simulink model "sin_wave_demodulate"  (R2023b)
settings: Solver=VariableStepAuto  StartTime=0.0  StopTime=0.15  RelTol=1e-3
PreLoadFcn:
  | clear all;
  | 
  | fs = 1e6
InitFcn:
  | fs = 1e6
libraries: hdlBasic x33, hdlsllib x3, dspsrcs4 x2, simulink x1, vmcUtilities x1
settings Model: Creator=David Northcote  LastModifiedBy=clb20123
settings SolverCC: AlgebraicLoopSolver=TrustRegion
settings DataIOCC: ReturnWorkspaceOutputs=off
settings DebuggingCC: UnconnectedInputMsg=warning  UnconnectedOutputMsg=warning  UnconnectedLineMsg=warning  ArithmeticOperatorsInVariantConditions=warning
settings ModelReferenceCC: EnableRefExpFcnMdlSchedulingChecks=on
settings SFSimCC: SimUseLocalCustomCode=off  CustomCodeUndefinedFunction=UseInterfaceOnly
settings RTWCC: RTWUseLocalCustomCode=off

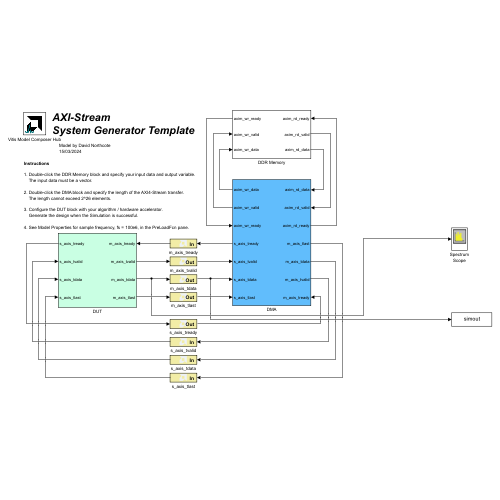
[thumbnail: Simulink's stored preview of the top-level diagram]
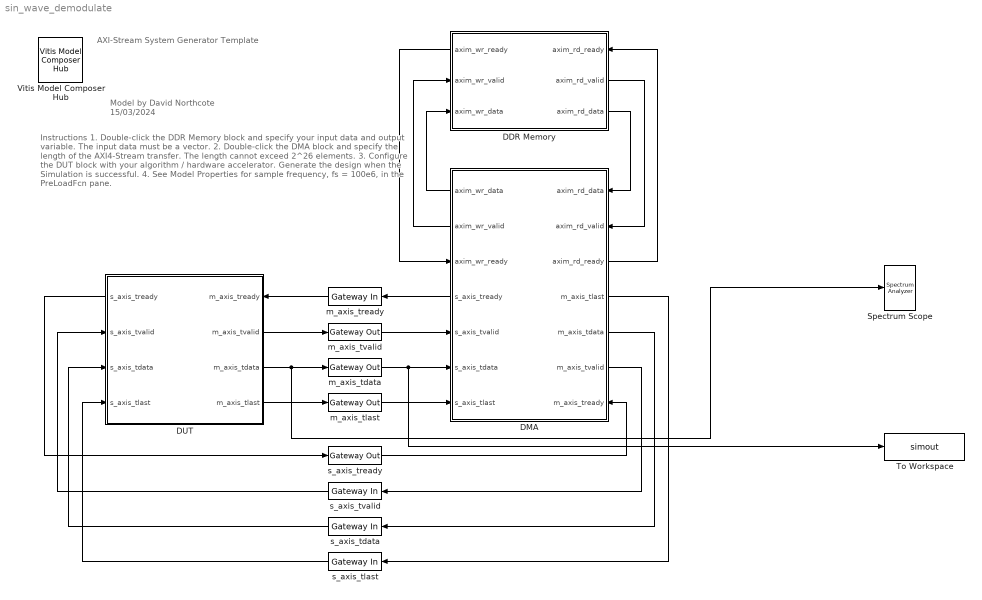
== system sin_wave_demodulate ==
  note: Instructions
      |
      | 1. Double-click the DDR Memory block and specify your input data and output variable.
      | The input data must be a vector.
      |
      | 2. Double-click the DMA block and specify the length of the AXI4-Stream transfer.
      | The length cannot exceed 2^26 elements.
      |
      | 3. Configure the DUT block with your algorithm / hardware accelerator.
      | Generate the design when the Simulation is successful.
      |
      | 4. See Model Properties for sample frequency, fs = 100e6, in the PreLoadFcn pane.
  note: Model by David Northcote
      | 15/03/2024
  note: AXI-Stream
      | System Generator Template
  DDR Memory : Subsystem  mask{bufferOut=[1 1 1 1 1 1 1 1 1 1 1 1 1 1], dtype=uint32, outVar='bufferIn'}
      mask prompts: bufferOut "Data to be sent:"; dtype "Data type:"; outVar "Output variable name:"
      mask init:
      | dtypeStr = get_param(gcb, 'dtype');
      | outVarStr = get_param(gcb, 'outVar');
      | set_param([gcb, '/Buffer In/To Workspace'], 'VariableName', outVar)
      settings: PortSchema="{\"entries\":[{\"content\":{\"sides\":[{\"content\":{\"connectorIds\":[\"Out3\",\"In1\",\"In2\"]},\"type\":\"ConnectorPlacement.EquallySpacedRectSide\",\"uuid\":\"10820561-fcd3-42da-ac38-14c6f993f770\"},{\"content\":{\"connectorIds\":[\"In3\",\"Out1\",\"Out2\"],\"side\":\"RIGHT\"},\"type\":\"ConnectorPlacement.EquallySpacedRectSide\",\"uuid\":\"072276f7-1cf8-495f-bb0a-1bca7e8326ea\"},{\"content\":{\"connectorIds\":[],\"side\":\"TOP\"},\"type\":\"ConnectorPlacement.EquallySpacedRectSide\",\"uuid\":\"f5b81d71-f8e7-451c-95ca-ef44dafc9f7a\"}]},\"type\":\"ConnectorPlacement.EquallySpacedConnector\",\"uuid\":\"59ea238c-ea64-4381-b9ec-a479227d5ff5\"}],\"packageUris\":[\"http://schema.mathworks.com/mf0/Connector/19700101\"],\"version\":\"1.0\"}"
      mask TypeOptions dtype: uint32 | int32
      mask DialogControl DescGroupVar Prompt: DDR Memory
      mask DialogControl DescTextVar Prompt: Block simulating a DDR memory controller.
      mask DialogControl ParameterGroupVar Prompt: MM2S
      mask DialogControl Container4 Prompt: S2MM
  DMA : Subsystem  mask{N=32}
      mask prompts: N "Length of data:"
      settings: PortSchema="{\"entries\":[{\"content\":{\"sides\":[{\"content\":{\"connectorIds\":[\"Out5\",\"Out6\",\"In1\",\"Out7\",\"In2\",\"In3\",\"In4\"]},\"type\":\"ConnectorPlacement.EquallySpacedRectSide\",\"uuid\":\"c102abcb-2e00-4fd7-85df-5b9b0b898bd0\"},{\"content\":{\"connectorIds\":[\"In5\",\"In6\",\"Out1\",\"Out2\",\"Out3\",\"Out4\",\"In7\"],\"side\":\"RIGHT\"},\"type\":\"ConnectorPlacement.EquallySpacedRectSide\",\"uuid\":\"9e178eef-1e1d-41e3-971e-2eb7c6a5387e\"},{\"content\":{\"connectorIds\":[],\"side\":\"TOP\"},\"type\":\"ConnectorPlacement.EquallySpacedRectSide\",\"uuid\":\"12cf59e0-f07a-41d8-b174-5a1eb72b1624\"},{\"content\":{\"connectorIds\":[],\"side\":\"BOTTOM\"},\"type\":\"ConnectorPlacement.EquallySpacedRectSide\",\"uuid\":\"a47cc6bb-72ec-4c9c-b625-c22428f6e2e0\"}]},\"type\":\"ConnectorPlacement.EquallySpacedConnector\",\"uuid\":\"cad21ed4-9065-49eb-a891-849a058d114a\"}],\"packageUris\":[\"http://schema.mathworks.com/mf0/Connector/19700101\"],\"version\":\"1.0\"}"
      mask DialogControl DescGroupVar Prompt: AXI DMA
      mask DialogControl DescTextVar Prompt: Block simulating an AXI DMA.
      mask DialogControl ParameterGroupVar Prompt: Main
  DUT : Subsystem
      settings: PortSchema="{\"entries\":[{\"content\":{\"sides\":[{\"content\":{\"connectorIds\":[\"Out4\",\"In1\",\"In2\",\"In3\"]},\"type\":\"ConnectorPlacement.EquallySpacedRectSide\",\"uuid\":\"c102abcb-2e00-4fd7-85df-5b9b0b898bd0\"},{\"content\":{\"connectorIds\":[\"In4\",\"Out1\",\"Out2\",\"Out3\"],\"side\":\"RIGHT\"},\"type\":\"ConnectorPlacement.EquallySpacedRectSide\",\"uuid\":\"9e178eef-1e1d-41e3-971e-2eb7c6a5387e\"},{\"content\":{\"connectorIds\":[],\"side\":\"TOP\"},\"type\":\"ConnectorPlacement.EquallySpacedRectSide\",\"uuid\":\"12cf59e0-f07a-41d8-b174-5a1eb72b1624\"}]},\"type\":\"ConnectorPlacement.EquallySpacedConnector\",\"uuid\":\"cad21ed4-9065-49eb-a891-849a058d114a\"}],\"packageUris\":[\"http://schema.mathworks.com/mf0/Connector/19700101\"],\"version\":\"1.0\"}"
  Spectrum Scope : SpectrumAnalyzer  WindowPosition=[182.000000,-8.000000,1444.000000,881.000000,]  ScopeFrameLocation=window  SpectrumType=Power density  Method=Welch  SampleRate=48000  PlotAsTwoSidedSpectrum=off  AxesScaling=Manual  FrequencySpan=Start and stop frequencies  Span=24000  CenterFrequency=12000  StartFrequency=0  StopFrequency=fs/2  FrequencyResolutionMethod=Window length  FFTLengthSource=Property  FFTLength=2048  WindowLength=2048  OverlapPercent=50  AveragingMethod=Running  SpectralAverages=2  SpectrumUnits=dBW/Hz  YLabel=Magnitude  YLimits=[-1013.06950271,305.05930835]  SelectedToolstripTab=spectrumAnalyzerToolstrip.measurementsTab  DefaultConfigurationName=spbscopes.SpectrumAnalyzerBlockCfg  IsFrequencyInputMode=0  FrequencyVectorPort=0  FrequencyVectorFromPort=0  FrequencyInputRBWPort=0  FrequencyInputRBWFromPort=0  SegLen=2048
  To Workspace : ToWorkspace  VariableName=simout  SaveFormat=Timeseries  SampleTime=-1
  Vitis Model Composer Hub : vmcUtilities/Vitis Model Composer Hub  Tag=genX  CodeGeneration=off  SubsystemName=sin_wave_modulate  CompilationType=HDLCompilation  ExportTypeV2=IP Catalog  TargetDirectory=./netlist  exportDesign=on  analyzeDesign=off  validateDesignOnHw=off  ExportType=System Generator  IpVendor=xilinx.com  IpLibrary=hls  IpVersion=1.0  IpHWLanguage=Verilog  AieCompilerOptions={}  AieSimulatorOptions={}  CreateTestbench=off  TestbenchStackSize=10  RunRtlSim=off  RunCSim=off  RunAieSim=off  AieSimTimeout=50000  RunAieSimProfiling=off  LaunchVitisAnalyzer=off  PlotOutput=off  RunX86Sim=off  X86SimTimeout=10  GenHwImage=off  GenLibadfXo=on  GenHwValidationCode=off  PlatformType=Not Specified  HwSystemType=Baremetal  HwValidationTarget=hw  ProjDevice=xczu43dr-ffve1156-2-e  ProjDevicePart=xczu43dr-ffve1156-2-e  SamplePeriod=-1  ClockFrequency=200  DataPathParallelism=1  xilinxfamily=zynquplusRFSOC  part=xczu43dr  speed=-2-e  package=ffve1156  directory=./netlist\ip\sin_wave_modulate\src  testbench=off  incr_netlist=off  synthesis_tool=Vivado  clock_wrapper=Clock Enables  dbl_ovrd=According to Block Masks  dcm_input_clock_period=10  sysclk_period=10  simulink_period=1/fs  eval_field=0  IPInfoJsonString="{\"HDLSubsystem\":{\"SubsystemName\":\"AXI_Overtone\",\"IPName\":\"axi_stream_template\",\"IPLibrary\":\"SysGen\",\"IPVendor\":\"strath.ac.uk\",\"IPVersion\":\"1.0\",\"TargetDirectory\":\"./netlist\",\"SubsystemDir\":\"./netlist\\\\ip\\\\AXI_Overtone\"},\"SubsystemTag\":\"HDLNode\"}"  LogFileName=''  NThreads=4
  m_axis_tdata : hdlBasic/Gateway Out  inherit_from_input=on  hdl_port=on  rows=1  columns=1  UseAsDAC=off  DACChannel='1'  interface=None  automatic_assignment=on  address_offset=hex2dec('00')  intf_name=''  intf_description=''  timing_constraint=None  locs_specified=off  LOCs={}  io_standard={}  XmcBlockStatus=1  maskContainerNames=group4  block_type=gatewayout  block_config=sysgen:gateway_out_config  block_width_w=590  block_height_w=620  block_width=620  block_height=750
  m_axis_tlast : hdlBasic/Gateway Out  inherit_from_input=on  hdl_port=on  rows=1  columns=1  UseAsDAC=off  DACChannel='1'  interface=None  automatic_assignment=on  address_offset=hex2dec('00')  intf_name=''  intf_description=''  timing_constraint=None  locs_specified=off  LOCs={}  io_standard={}  XmcBlockStatus=1  maskContainerNames=group4  block_type=gatewayout  block_config=sysgen:gateway_out_config  block_width_w=590  block_height_w=620  block_width=620  block_height=750
  m_axis_tready : hdlBasic/Gateway In  gui_display_data_type=Boolean  arith_type=Boolean  n_bits=16  bin_pt=14  preci_type=Single  exp_width=8  frac_width=24  rows=1  columns=1  quantization="Round  (unbiased: +/- Inf)"  overflow=Saturate  period=1/fs  UseAsADC=off  ADCChannel='1'  interface=None  automatic_assignment=on  address_offset=hex2dec('00')  intf_name=''  intf_description=''  default_value=0  timing_constraint=None  locs_specified=off  LOCs={}  io_standard={}  inherit_from_input=off  hdl_port=on  XmcBlockStatus=1  maskContainerNames=group4  block_type=gatewayin  block_config=sysgen:gateway_in_config  block_width_w=590  block_height_w=620  block_width=640  block_height=850
  m_axis_tvalid : hdlBasic/Gateway Out  inherit_from_input=on  hdl_port=on  rows=1  columns=1  UseAsDAC=off  DACChannel='1'  interface=None  automatic_assignment=on  address_offset=hex2dec('00')  intf_name=''  intf_description=''  timing_constraint=None  locs_specified=off  LOCs={}  io_standard={}  XmcBlockStatus=1  maskContainerNames=group4  block_type=gatewayout  block_config=sysgen:gateway_out_config  block_width_w=590  block_height_w=620  block_width=620  block_height=750
  s_axis_tdata : hdlBasic/Gateway In  gui_display_data_type=Fixed-point  arith_type=Unsigned  n_bits=1  bin_pt=0  preci_type=Single  exp_width=8  frac_width=24  rows=1  columns=1  quantization="Round  (unbiased: +/- Inf)"  overflow=Saturate  period=1/fs  UseAsADC=off  ADCChannel='1'  interface=None  automatic_assignment=on  address_offset=hex2dec('00')  intf_name=''  intf_description=''  default_value=0  timing_constraint=None  locs_specified=off  LOCs={}  io_standard={}  inherit_from_input=off  hdl_port=on  XmcBlockStatus=1  maskContainerNames=group4  block_type=gatewayin  block_config=sysgen:gateway_in_config  block_width_w=590  block_height_w=620  block_width=640  block_height=850
  s_axis_tlast : hdlBasic/Gateway In  gui_display_data_type=Boolean  arith_type=Boolean  n_bits=16  bin_pt=14  preci_type=Single  exp_width=8  frac_width=24  rows=1  columns=1  quantization="Round  (unbiased: +/- Inf)"  overflow=Saturate  period=1/fs  UseAsADC=off  ADCChannel='1'  interface=None  automatic_assignment=on  address_offset=hex2dec('00')  intf_name=''  intf_description=''  default_value=0  timing_constraint=None  locs_specified=off  LOCs={}  io_standard={}  inherit_from_input=off  hdl_port=on  XmcBlockStatus=1  maskContainerNames=group4  block_type=gatewayin  block_config=sysgen:gateway_in_config  block_width_w=590  block_height_w=620  block_width=640  block_height=850
  s_axis_tready : hdlBasic/Gateway Out  inherit_from_input=on  hdl_port=on  rows=1  columns=1  UseAsDAC=off  DACChannel='1'  interface=None  automatic_assignment=on  address_offset=hex2dec('00')  intf_name=''  intf_description=''  timing_constraint=None  locs_specified=off  LOCs={}  io_standard={}  XmcBlockStatus=1  maskContainerNames=group4  block_type=gatewayout  block_config=sysgen:gateway_out_config  block_width_w=590  block_height_w=620  block_width=620  block_height=750
  s_axis_tvalid : hdlBasic/Gateway In  gui_display_data_type=Boolean  arith_type=Boolean  n_bits=16  bin_pt=14  preci_type=Single  exp_width=8  frac_width=24  rows=1  columns=1  quantization="Round  (unbiased: +/- Inf)"  overflow=Saturate  period=1/fs  UseAsADC=off  ADCChannel='1'  interface=None  automatic_assignment=on  address_offset=hex2dec('00')  intf_name=''  intf_description=''  default_value=0  timing_constraint=None  locs_specified=off  LOCs={}  io_standard={}  inherit_from_input=off  hdl_port=on  XmcBlockStatus=1  maskContainerNames=group4  block_type=gatewayin  block_config=sysgen:gateway_in_config  block_width_w=590  block_height_w=620  block_width=640  block_height=850
  wires:
  s_axis_tvalid/1 -> DUT/1(s_axis_tvalid)
  s_axis_tdata/1 -> DUT/2(s_axis_tdata)
  s_axis_tlast/1 -> DUT/3(s_axis_tlast)
  m_axis_tready/1 -> DUT/4(m_axis_tready)
  DUT/4(s_axis_tready) -> s_axis_tready/1
  DUT/2(m_axis_tdata) -> Spectrum Scope/1, m_axis_tdata/1
  DUT/1(m_axis_tvalid) -> m_axis_tvalid/1
  DUT/3(m_axis_tlast) -> m_axis_tlast/1
  s_axis_tready/1 -> DMA/7(m_axis_tready)
  DMA/4(m_axis_tvalid) -> s_axis_tvalid/1
  DMA/3(m_axis_tdata) -> s_axis_tdata/1
  DMA/2(m_axis_tlast) -> s_axis_tlast/1
  DMA/7(s_axis_tready) -> m_axis_tready/1
  m_axis_tvalid/1 -> DMA/2(s_axis_tvalid)
  m_axis_tdata/1 -> To Workspace/1, DMA/3(s_axis_tdata)
  m_axis_tlast/1 -> DMA/4(s_axis_tlast)
  DMA/1(axim_rd_ready) -> DDR Memory/3(axim_rd_ready)
  DDR Memory/1(axim_rd_valid) -> DMA/6(axim_rd_valid)
  DDR Memory/2(axim_rd_data) -> DMA/5(axim_rd_data)
  DDR Memory/3(axim_wr_ready) -> DMA/1(axim_wr_ready)
  DMA/6(axim_wr_valid) -> DDR Memory/1(axim_wr_valid)
  DMA/5(axim_wr_data) -> DDR Memory/2(axim_wr_data)

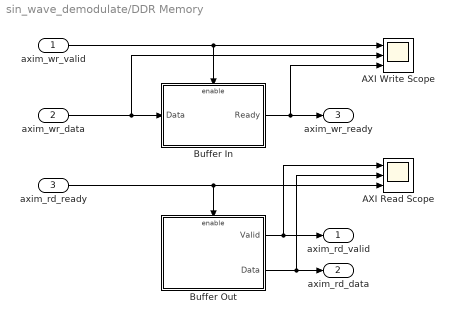
== system sin_wave_demodulate/DDR Memory ==
  axim_wr_valid : Inport
  axim_wr_data : Inport  Port=2
  axim_rd_ready : Inport  Port=3
  AXI Read Scope : Scope  NumInputPorts=3
  AXI Write Scope : Scope  NumInputPorts=3
  Buffer In : Subsystem
  Buffer Out : Subsystem
  axim_rd_valid : Outport
  axim_rd_data : Outport  Port=2
  axim_wr_ready : Outport  Port=3
  wires:
  Buffer Out/1(Valid) -> AXI Read Scope/1, axim_rd_valid/1
  Buffer Out/2(Data) -> AXI Read Scope/2, axim_rd_data/1
  axim_rd_ready/1 -> Buffer Out/Enable, AXI Read Scope/3
  axim_wr_data/1 -> AXI Write Scope/2, Buffer In/1(Data)
  Buffer In/1(Ready) -> AXI Write Scope/3, axim_wr_ready/1
  axim_wr_valid/1 -> Buffer In/Enable, AXI Write Scope/1

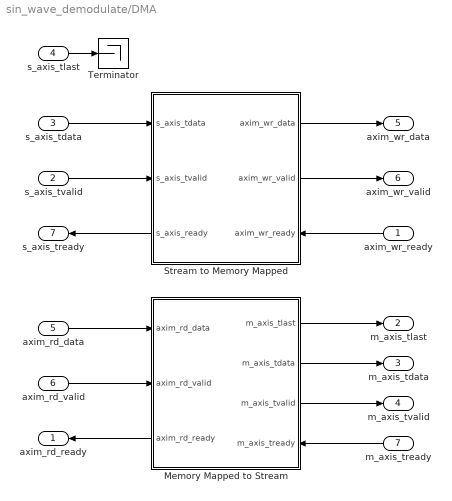
== system sin_wave_demodulate/DMA ==
  axim_wr_ready : Inport
  s_axis_tvalid : Inport  Port=2
  s_axis_tdata : Inport  Port=3
  s_axis_tlast : Inport  Port=4
  axim_rd_data : Inport  Port=5
  axim_rd_valid : Inport  Port=6
  m_axis_tready : Inport  Port=7
  Memory Mapped to Stream : Subsystem
      settings: PortSchema="{\"entries\":[{\"content\":{\"sides\":[{\"content\":{\"connectorIds\":[\"In1\",\"In2\",\"Out4\"]},\"type\":\"ConnectorPlacement.EquallySpacedRectSide\",\"uuid\":\"10820561-fcd3-42da-ac38-14c6f993f770\"},{\"content\":{\"connectorIds\":[\"Out1\",\"Out2\",\"Out3\",\"In3\"],\"side\":\"RIGHT\"},\"type\":\"ConnectorPlacement.EquallySpacedRectSide\",\"uuid\":\"072276f7-1cf8-495f-bb0a-1bca7e8326ea\"},{\"content\":{\"connectorIds\":[],\"side\":\"TOP\"},\"type\":\"ConnectorPlacement.EquallySpacedRectSide\",\"uuid\":\"f5b81d71-f8e7-451c-95ca-ef44dafc9f7a\"}]},\"type\":\"ConnectorPlacement.EquallySpacedConnector\",\"uuid\":\"59ea238c-ea64-4381-b9ec-a479227d5ff5\"}],\"packageUris\":[\"http://schema.mathworks.com/mf0/Connector/19700101\"],\"version\":\"1.0\"}"
  Stream to Memory Mapped : Subsystem
      settings: PortSchema="{\"entries\":[{\"content\":{\"sides\":[{\"content\":{\"connectorIds\":[\"In1\",\"In2\",\"Out3\"]},\"type\":\"ConnectorPlacement.EquallySpacedRectSide\",\"uuid\":\"10820561-fcd3-42da-ac38-14c6f993f770\"},{\"content\":{\"connectorIds\":[\"Out1\",\"Out2\",\"In3\"],\"side\":\"RIGHT\"},\"type\":\"ConnectorPlacement.EquallySpacedRectSide\",\"uuid\":\"072276f7-1cf8-495f-bb0a-1bca7e8326ea\"},{\"content\":{\"connectorIds\":[],\"side\":\"TOP\"},\"type\":\"ConnectorPlacement.EquallySpacedRectSide\",\"uuid\":\"f5b81d71-f8e7-451c-95ca-ef44dafc9f7a\"}]},\"type\":\"ConnectorPlacement.EquallySpacedConnector\",\"uuid\":\"59ea238c-ea64-4381-b9ec-a479227d5ff5\"}],\"packageUris\":[\"http://schema.mathworks.com/mf0/Connector/19700101\"],\"version\":\"1.0\"}"
  Terminator : Terminator
  axim_rd_ready : Outport
  m_axis_tlast : Outport  Port=2  VectorParamsAs1DForOutWhenUnconnected=off
  m_axis_tdata : Outport  Port=3  VectorParamsAs1DForOutWhenUnconnected=off
  m_axis_tvalid : Outport  Port=4  VectorParamsAs1DForOutWhenUnconnected=off
  axim_wr_data : Outport  Port=5
  axim_wr_valid : Outport  Port=6
  s_axis_tready : Outport  Port=7  VectorParamsAs1DForOutWhenUnconnected=off
  wires:
  m_axis_tready/1 -> Memory Mapped to Stream/3(m_axis_tready)
  Memory Mapped to Stream/1(m_axis_tlast) -> m_axis_tlast/1
  Memory Mapped to Stream/2(m_axis_tdata) -> m_axis_tdata/1
  Memory Mapped to Stream/3(m_axis_tvalid) -> m_axis_tvalid/1
  s_axis_tvalid/1 -> Stream to Memory Mapped/2(s_axis_tvalid)
  s_axis_tdata/1 -> Stream to Memory Mapped/1(s_axis_tdata)
  Stream to Memory Mapped/3(s_axis_ready) -> s_axis_tready/1
  s_axis_tlast/1 -> Terminator/1
  Stream to Memory Mapped/1(axim_wr_data) -> axim_wr_data/1
  Stream to Memory Mapped/2(axim_wr_valid) -> axim_wr_valid/1
  axim_wr_ready/1 -> Stream to Memory Mapped/3(axim_wr_ready)
  Memory Mapped to Stream/4(axim_rd_ready) -> axim_rd_ready/1
  axim_rd_data/1 -> Memory Mapped to Stream/1(axim_rd_data)
  axim_rd_valid/1 -> Memory Mapped to Stream/2(axim_rd_valid)

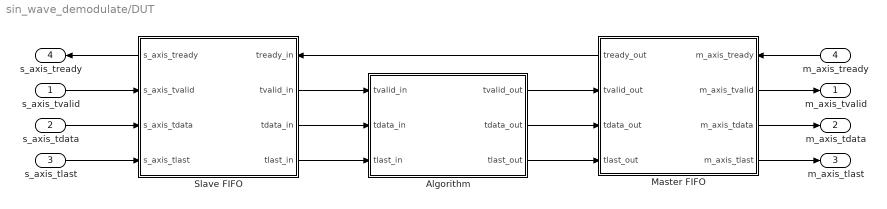
== system sin_wave_demodulate/DUT ==
  s_axis_tvalid : Inport
  s_axis_tdata : Inport  Port=2
  s_axis_tlast : Inport  Port=3
  m_axis_tready : Inport  Port=4
  Algorithm : Subsystem
  Master FIFO : Subsystem
      settings: PortSchema="{\"entries\":[{\"content\":{\"sides\":[{\"content\":{\"connectorIds\":[\"Out4\",\"In1\",\"In2\",\"In3\"]},\"type\":\"ConnectorPlacement.EquallySpacedRectSide\",\"uuid\":\"10820561-fcd3-42da-ac38-14c6f993f770\"},{\"content\":{\"connectorIds\":[\"In4\",\"Out1\",\"Out2\",\"Out3\"],\"side\":\"RIGHT\"},\"type\":\"ConnectorPlacement.EquallySpacedRectSide\",\"uuid\":\"072276f7-1cf8-495f-bb0a-1bca7e8326ea\"},{\"content\":{\"connectorIds\":[],\"side\":\"TOP\"},\"type\":\"ConnectorPlacement.EquallySpacedRectSide\",\"uuid\":\"f5b81d71-f8e7-451c-95ca-ef44dafc9f7a\"}]},\"type\":\"ConnectorPlacement.EquallySpacedConnector\",\"uuid\":\"59ea238c-ea64-4381-b9ec-a479227d5ff5\"}],\"packageUris\":[\"http://schema.mathworks.com/mf0/Connector/19700101\"],\"version\":\"1.0\"}"
  Slave FIFO : Subsystem
      settings: PortSchema="{\"entries\":[{\"content\":{\"sides\":[{\"content\":{\"connectorIds\":[\"Out4\",\"In1\",\"In2\",\"In3\"]},\"type\":\"ConnectorPlacement.EquallySpacedRectSide\",\"uuid\":\"10820561-fcd3-42da-ac38-14c6f993f770\"},{\"content\":{\"connectorIds\":[\"In4\",\"Out1\",\"Out2\",\"Out3\"],\"side\":\"RIGHT\"},\"type\":\"ConnectorPlacement.EquallySpacedRectSide\",\"uuid\":\"072276f7-1cf8-495f-bb0a-1bca7e8326ea\"},{\"content\":{\"connectorIds\":[],\"side\":\"TOP\"},\"type\":\"ConnectorPlacement.EquallySpacedRectSide\",\"uuid\":\"f5b81d71-f8e7-451c-95ca-ef44dafc9f7a\"}]},\"type\":\"ConnectorPlacement.EquallySpacedConnector\",\"uuid\":\"59ea238c-ea64-4381-b9ec-a479227d5ff5\"}],\"packageUris\":[\"http://schema.mathworks.com/mf0/Connector/19700101\"],\"version\":\"1.0\"}"
  m_axis_tvalid : Outport  VectorParamsAs1DForOutWhenUnconnected=off
  m_axis_tdata : Outport  Port=2  VectorParamsAs1DForOutWhenUnconnected=off
  m_axis_tlast : Outport  Port=3  VectorParamsAs1DForOutWhenUnconnected=off
  s_axis_tready : Outport  Port=4  VectorParamsAs1DForOutWhenUnconnected=off
  wires:
  Master FIFO/1(m_axis_tvalid) -> m_axis_tvalid/1
  Master FIFO/2(m_axis_tdata) -> m_axis_tdata/1
  Master FIFO/3(m_axis_tlast) -> m_axis_tlast/1
  Algorithm/1(tvalid_out) -> Master FIFO/1(tvalid_out)
  Algorithm/2(tdata_out) -> Master FIFO/2(tdata_out)
  Algorithm/3(tlast_out) -> Master FIFO/3(tlast_out)
  s_axis_tvalid/1 -> Slave FIFO/1(s_axis_tvalid)
  s_axis_tdata/1 -> Slave FIFO/2(s_axis_tdata)
  s_axis_tlast/1 -> Slave FIFO/3(s_axis_tlast)
  Slave FIFO/1(tvalid_in) -> Algorithm/1(tvalid_in)
  Slave FIFO/2(tdata_in) -> Algorithm/2(tdata_in)
  Slave FIFO/3(tlast_in) -> Algorithm/3(tlast_in)
  Slave FIFO/4(s_axis_tready) -> s_axis_tready/1
  m_axis_tready/1 -> Master FIFO/4(m_axis_tready)
  Master FIFO/4(tready_out) -> Slave FIFO/4(tready_in)

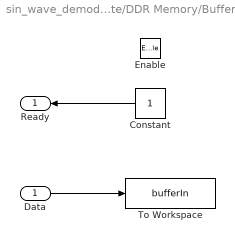
== system sin_wave_demodulate/DDR Memory/Buffer In ==
  Data : Inport
  Enable : EnablePort
  Constant : Constant  OutDataTypeStr=boolean  SampleTime=-1
  To Workspace : ToWorkspace  VariableName=bufferIn  SampleTime=-1
  Ready : Outport
  wires:
  Data/1 -> To Workspace/1
  Constant/1 -> Ready/1

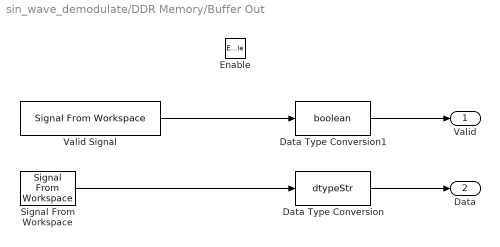
== system sin_wave_demodulate/DDR Memory/Buffer Out ==
  Enable : EnablePort
  Data Type Conversion : DataTypeConversion  OutDataTypeStr=dtypeStr  SaturateOnIntegerOverflow=off  RndMeth=Floor
  Data Type Conversion1 : DataTypeConversion  OutDataTypeStr=boolean  SaturateOnIntegerOverflow=off  RndMeth=Floor
  Signal From Workspace : dspsrcs4/Signal From Workspace  X=bufferOut  Ts=1/fs  nsamps=1  OutputAfterFinalValue=Setting to zero  ignoreOrWarnInputAndFrameLengths=off  OutputFrames=off
  Valid Signal : dspsrcs4/Signal From Workspace  X=ones(1, length(bufferOut))  Ts=1/fs  nsamps=1  OutputAfterFinalValue=Setting to zero  ignoreOrWarnInputAndFrameLengths=off  OutputFrames=off
  Valid : Outport
  Data : Outport  Port=2
  wires:
  Signal From Workspace/1 -> Data Type Conversion/1
  Data Type Conversion/1 -> Data/1
  Valid Signal/1 -> Data Type Conversion1/1
  Data Type Conversion1/1 -> Valid/1

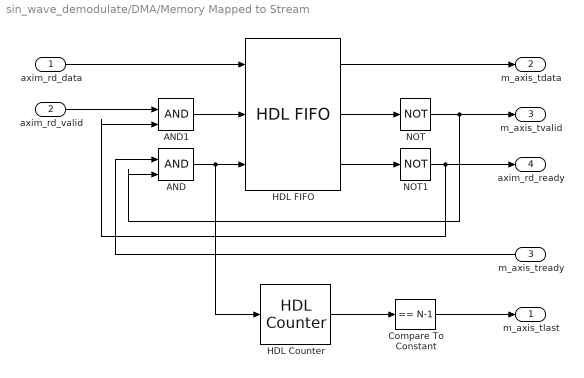
== system sin_wave_demodulate/DMA/Memory Mapped to Stream ==
  axim_rd_data : Inport
  axim_rd_valid : Inport  Port=2
  m_axis_tready : Inport  Port=3
  AND : Logic  IconShape=distinctive  AllPortsSameDT=off  OutDataTypeStr=boolean
  AND1 : Logic  IconShape=distinctive  AllPortsSameDT=off  OutDataTypeStr=boolean
  Compare To Constant : simulink/Logic and Bit Operations/Compare To Constant  relop===  const=N-1  OutDataTypeStr=boolean
  HDL Counter : hdlsllib/Sources/HDL Counter  CountType=Count limited  CountInit=0  CountStep=1  CountMax=N-1  CountFromType=Initial value  CountFrom=0  CountResetPort=off  CountLoadPort=off  CountEnbPort=on  CountDirPort=off  CountHitOutputPort=off  CountDataType=Unsigned  CountWordLen=ceil(log2(N))  CountFracLen=0  CountSampTime=1
  HDL FIFO : hdlsllib/HDL RAMs/HDL FIFO  fifo_size=16  mode=FWFT  ratio=1  push_msg=Warning  pop_msg=Warning  show_empty=on  show_full=on  show_num=off  LabelModeActiveChoice_Mode=FWFT  rst_port=off
  NOT : Logic  Operator=NOT  IconShape=distinctive  AllPortsSameDT=off  OutDataTypeStr=boolean
  NOT1 : Logic  Operator=NOT  IconShape=distinctive  AllPortsSameDT=off  OutDataTypeStr=boolean
  m_axis_tlast : Outport  VectorParamsAs1DForOutWhenUnconnected=off
  m_axis_tdata : Outport  Port=2  VectorParamsAs1DForOutWhenUnconnected=off
  m_axis_tvalid : Outport  Port=3  VectorParamsAs1DForOutWhenUnconnected=off
  axim_rd_ready : Outport  Port=4  VectorParamsAs1DForOutWhenUnconnected=off
  wires:
  NOT/1 -> m_axis_tvalid/1, AND/2
  HDL Counter/1 -> Compare To Constant/1
  m_axis_tready/1 -> AND/1
  AND/1 -> HDL Counter/1, HDL FIFO/3
  Compare To Constant/1 -> m_axis_tlast/1
  HDL FIFO/2 -> NOT/1
  AND1/1 -> HDL FIFO/2
  HDL FIFO/1 -> m_axis_tdata/1
  HDL FIFO/3 -> NOT1/1
  NOT1/1 -> AND1/2, axim_rd_ready/1
  axim_rd_valid/1 -> AND1/1
  axim_rd_data/1 -> HDL FIFO/1

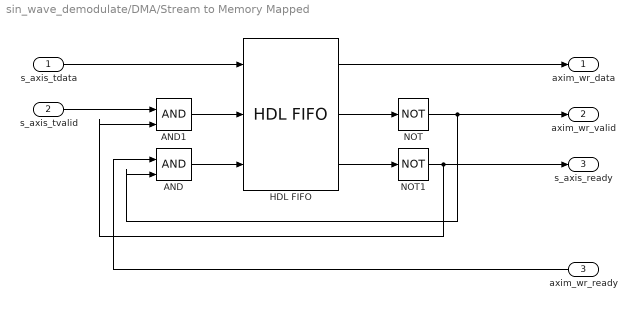
== system sin_wave_demodulate/DMA/Stream to Memory Mapped ==
  s_axis_tdata : Inport
  s_axis_tvalid : Inport  Port=2
  axim_wr_ready : Inport  Port=3
  AND : Logic  IconShape=distinctive  AllPortsSameDT=off  OutDataTypeStr=boolean
  AND1 : Logic  IconShape=distinctive  AllPortsSameDT=off  OutDataTypeStr=boolean
  HDL FIFO : hdlsllib/HDL RAMs/HDL FIFO  fifo_size=16  mode=FWFT  ratio=1  push_msg=Warning  pop_msg=Warning  show_empty=on  show_full=on  show_num=off  LabelModeActiveChoice_Mode=FWFT  rst_port=off
  NOT : Logic  Operator=NOT  IconShape=distinctive  AllPortsSameDT=off  OutDataTypeStr=boolean
  NOT1 : Logic  Operator=NOT  IconShape=distinctive  AllPortsSameDT=off  OutDataTypeStr=boolean
  axim_wr_data : Outport  VectorParamsAs1DForOutWhenUnconnected=off
  axim_wr_valid : Outport  Port=2  VectorParamsAs1DForOutWhenUnconnected=off
  s_axis_ready : Outport  Port=3  VectorParamsAs1DForOutWhenUnconnected=off
  wires:
  s_axis_tvalid/1 -> AND1/1
  HDL FIFO/3 -> NOT1/1
  HDL FIFO/1 -> axim_wr_data/1
  AND1/1 -> HDL FIFO/2
  HDL FIFO/2 -> NOT/1
  AND/1 -> HDL FIFO/3
  axim_wr_ready/1 -> AND/1
  NOT/1 -> AND/2, axim_wr_valid/1
  s_axis_tdata/1 -> HDL FIFO/1
  NOT1/1 -> s_axis_ready/1, AND1/2

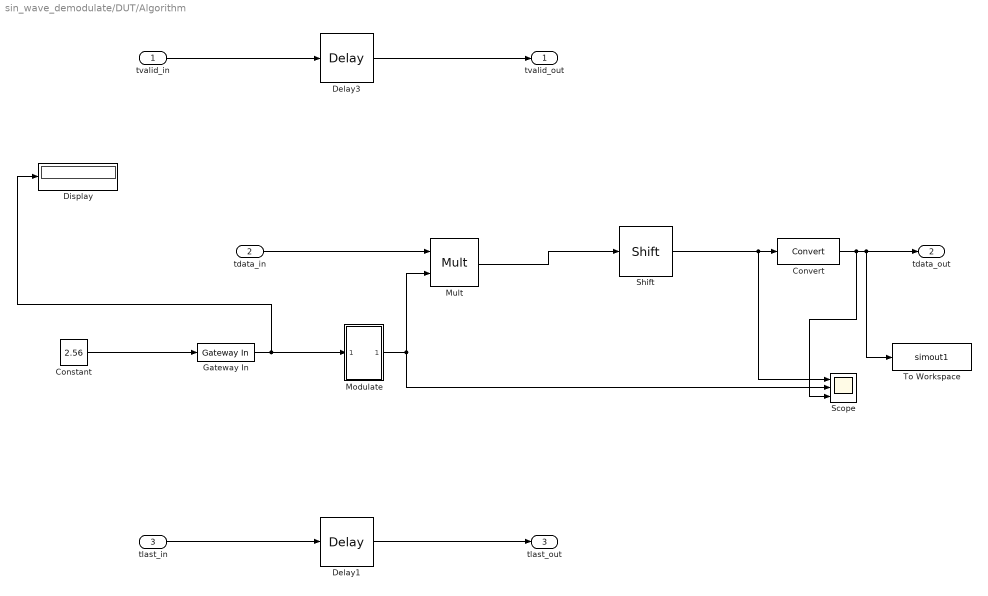
== system sin_wave_demodulate/DUT/Algorithm ==
  tvalid_in : Inport
  tdata_in : Inport  Port=2
  tlast_in : Inport  Port=3
  Constant : Constant  Value=2.56
  Convert : hdlBasic/Convert  gui_display_data_type=Fixed-point  arith_type=Unsigned  n_bits=32  bin_pt=0  float_type=Single  exp_bits=8  fraction_bits=24  quantization=Truncate  overflow=Wrap  en=off  latency=1  pipeline=off  XmcBlockStatus=1  maskContainerNames=group2  block_type=convert  block_config=sysgen:Convert_config  block_width=595  block_height=885
  Delay1 : hdlBasic/Delay  rst=off  en=off  latency=8  reg_retiming=off  XmcBlockStatus=1  maskContainerNames=group1  block_type=delay  block_config=sysgen:Delay_config
  Delay3 : hdlBasic/Delay  rst=off  en=off  latency=8  reg_retiming=off  XmcBlockStatus=1  maskContainerNames=group1  block_type=delay  block_config=sysgen:Delay_config
  Display : Display
  Gateway In : hdlBasic/Gateway In  gui_display_data_type=Fixed-point  arith_type=Signed (2's comp)  n_bits=16  bin_pt=12  preci_type=Single  exp_width=8  frac_width=24  rows=1  columns=1  quantization="Round  (unbiased: +/- Inf)"  overflow=Saturate  period=1/fs  UseAsADC=off  ADCChannel='1'  interface=None  automatic_assignment=on  address_offset=hex2dec('00')  intf_name=''  intf_description=''  default_value=0  timing_constraint=None  locs_specified=off  LOCs={}  io_standard={}  inherit_from_input=off  hdl_port=on  XmcBlockStatus=1  maskContainerNames=group4  block_type=gatewayin  block_config=sysgen:gateway_in_config  block_width_w=590  block_height_w=620  block_width=640  block_height=850
  Modulate : Subsystem
  Mult : hdlBasic/Mult  precision=User Defined  arith_type="Signed  (2's comp)"  n_bits=16  bin_pt=14  quantization=Truncate  overflow=Wrap  en=off  latency=3  use_behavioral_HDL=off  opt=Speed  use_embedded=on  optimum_pipeline=off  pipeline=on  use_rpm=on  placement_style=Triangular  XmcBlockStatus=1  maskContainerNames=group1  block_type=mult  block_config=sysgen:Mult_config  block_width=598  block_height=876
  Scope : Scope  NumInputPorts=3
  Shift : hdlBasic/Shift  shift_dir=Left  shift_bits=16  en=off  latency=1  precision=User Defined  arith_type="Signed  (2's comp)"  n_bits=32  bin_pt=0  quantization="Round  (unbiased: +/- Inf)"  overflow=Saturate  XmcBlockStatus=1  maskContainerNames=group2  block_type=shift  block_config=sysgen:Shift_config
  To Workspace : ToWorkspace  VariableName=simout1  SaveFormat=Timeseries  SampleTime=-1
  tvalid_out : Outport  VectorParamsAs1DForOutWhenUnconnected=off
  tdata_out : Outport  Port=2  VectorParamsAs1DForOutWhenUnconnected=off
  tlast_out : Outport  Port=3  VectorParamsAs1DForOutWhenUnconnected=off
  wires:
  tvalid_in/1 -> Delay3/1
  Delay3/1 -> tvalid_out/1
  Delay1/1 -> tlast_out/1
  tlast_in/1 -> Delay1/1
  Convert/1 -> Scope/3, tdata_out/1, To Workspace/1
  Shift/1 -> Scope/1, Convert/1
  tdata_in/1 -> Mult/1
  Mult/1 -> Shift/1
  Modulate/1(Out1) -> Mult/2, Scope/2
  Constant/1 -> Gateway In/1
  Gateway In/1 -> Display/1, Modulate/1(In1)

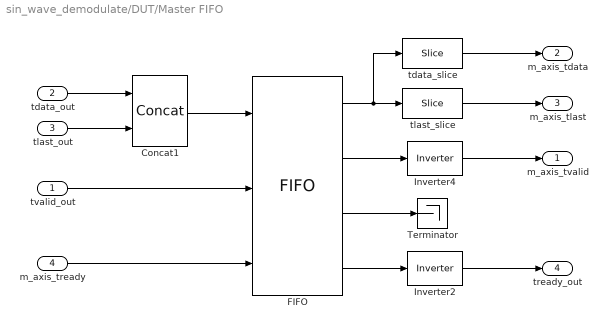
== system sin_wave_demodulate/DUT/Master FIFO ==
  tvalid_out : Inport
  tdata_out : Inport  Port=2
  tlast_out : Inport  Port=3
  m_axis_tready : Inport  Port=4
  Concat1 : hdlBasic/Concat  num_inputs=2  XmcBlockStatus=1  maskContainerNames=group1  block_type=concat  block_config=sysgen:Concat_config
  FIFO : hdlBasic/FIFO  mem_type=Block RAM  performance_options=First_Word_Fall_Through  embedded_registers=off  depth=1K  use_asym_data_widths=off  asym_read_width=32  percent_nbits=1  rst=off  rst_latency=2  en=off  use_dcount=off  use_percent_full_port=off  use_almost_empty=off  almost_empty_thresh=2  use_almost_full=on  use_rd_rst_busy=off  use_wr_rst_busy=off  almost_full_thresh=1000  almost_empty_offset=[]  almost_full_offset=[]  explicit_period=off  period=[]  store_only_valid=[]  init_zero=[]  simulation_type=fast_sim  XmcBlockStatus=1  maskContainerNames=tabcontainer1  block_type=fifo  block_config=sysgen:FIFO_config  block_width=538  block_height=997
      settings: infoedit=[]
  Inverter2 : hdlBasic/Inverter  en=off  latency=0  XmcBlockStatus=1  maskContainerNames=group2  block_type=inv  block_config=sysgen:Inverter_config
  Inverter4 : hdlBasic/Inverter  en=off  latency=0  XmcBlockStatus=1  maskContainerNames=group2  block_type=inv  block_config=sysgen:Inverter_config
  Terminator : Terminator
  tdata_slice : hdlBasic/Slice  nbits=1  boolean_output=off  mode=Two Bit Locations  bit1=0  base1=MSB of Input  bit0=1  base0=LSB of Input  XmcBlockStatus=1  maskContainerNames=group1  block_type=slice  block_config=sysgen:Slice_config
  tlast_slice : hdlBasic/Slice  nbits=1  boolean_output=on  mode=Two Bit Locations  bit1=0  base1=LSB of Input  bit0=0  base0=LSB of Input  XmcBlockStatus=1  maskContainerNames=group1  block_type=slice  block_config=sysgen:Slice_config
  m_axis_tvalid : Outport
  m_axis_tdata : Outport  Port=2
  m_axis_tlast : Outport  Port=3
  tready_out : Outport  Port=4
  wires:
  FIFO/4 -> Inverter2/1
  Inverter2/1 -> tready_out/1
  FIFO/2 -> Inverter4/1
  FIFO/1 -> tlast_slice/1, tdata_slice/1
  tlast_slice/1 -> m_axis_tlast/1
  tdata_slice/1 -> m_axis_tdata/1
  m_axis_tready/1 -> FIFO/3
  tvalid_out/1 -> FIFO/2
  Concat1/1 -> FIFO/1
  tdata_out/1 -> Concat1/1
  tlast_out/1 -> Concat1/2
  Inverter4/1 -> m_axis_tvalid/1
  FIFO/3 -> Terminator/1

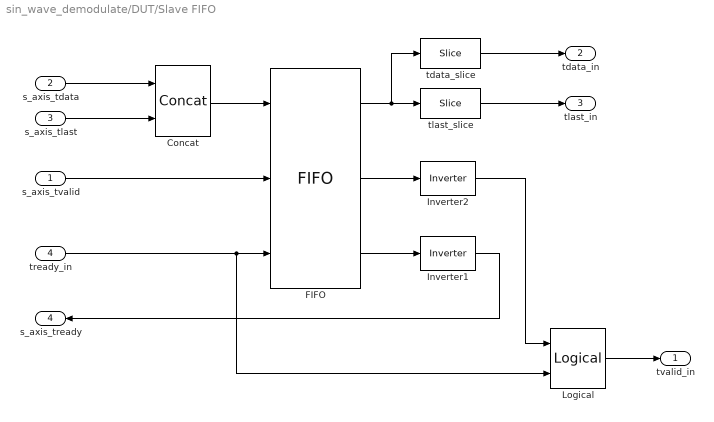
== system sin_wave_demodulate/DUT/Slave FIFO ==
  s_axis_tvalid : Inport
  s_axis_tdata : Inport  Port=2
  s_axis_tlast : Inport  Port=3
  tready_in : Inport  Port=4
  Concat : hdlBasic/Concat  num_inputs=2  XmcBlockStatus=1  maskContainerNames=group1  block_type=concat  block_config=sysgen:Concat_config
  FIFO : hdlBasic/FIFO  mem_type=Block RAM  performance_options=First_Word_Fall_Through  embedded_registers=off  depth=1K  use_asym_data_widths=off  asym_read_width=32  percent_nbits=1  rst=off  rst_latency=2  en=off  use_dcount=off  use_percent_full_port=off  use_almost_empty=off  almost_empty_thresh=2  use_almost_full=off  use_rd_rst_busy=off  use_wr_rst_busy=off  almost_full_thresh=14  almost_empty_offset=[]  almost_full_offset=[]  explicit_period=off  period=[]  store_only_valid=[]  init_zero=[]  simulation_type=fast_sim  XmcBlockStatus=1  maskContainerNames=tabcontainer1  block_type=fifo  block_config=sysgen:FIFO_config  block_width=538  block_height=997
      settings: infoedit=[]
  Inverter1 : hdlBasic/Inverter  en=off  latency=0  XmcBlockStatus=1  maskContainerNames=group2  block_type=inv  block_config=sysgen:Inverter_config
  Inverter2 : hdlBasic/Inverter  en=off  latency=0  XmcBlockStatus=1  maskContainerNames=group2  block_type=inv  block_config=sysgen:Inverter_config
  Logical : hdlBasic/Logical  logical_function=AND  inputs=2  en=off  latency=0  precision=Full  arith_type=Unsigned  n_bits=16  bin_pt=0  align_bp=on  overflow=[]  quantization=[]  XmcBlockStatus=1  maskContainerNames=tabcontainer1  block_type=logical  block_config=sysgen:Logical_config
  tdata_slice : hdlBasic/Slice  nbits=1  boolean_output=off  mode=Two Bit Locations  bit1=0  base1=MSB of Input  bit0=1  base0=LSB of Input  XmcBlockStatus=1  maskContainerNames=group1  block_type=slice  block_config=sysgen:Slice_config
  tlast_slice : hdlBasic/Slice  nbits=1  boolean_output=on  mode=Two Bit Locations  bit1=0  base1=LSB of Input  bit0=0  base0=LSB of Input  XmcBlockStatus=1  maskContainerNames=group1  block_type=slice  block_config=sysgen:Slice_config
  tvalid_in : Outport
  tdata_in : Outport  Port=2
  tlast_in : Outport  Port=3
  s_axis_tready : Outport  Port=4
  wires:
  FIFO/3 -> Inverter1/1
  s_axis_tvalid/1 -> FIFO/2
  tready_in/1 -> Logical/2, FIFO/3
  Concat/1 -> FIFO/1
  s_axis_tdata/1 -> Concat/1
  s_axis_tlast/1 -> Concat/2
  FIFO/1 -> tdata_slice/1, tlast_slice/1
  tlast_slice/1 -> tlast_in/1
  tdata_slice/1 -> tdata_in/1
  Inverter1/1 -> s_axis_tready/1
  FIFO/2 -> Inverter2/1
  Inverter2/1 -> Logical/1
  Logical/1 -> tvalid_in/1

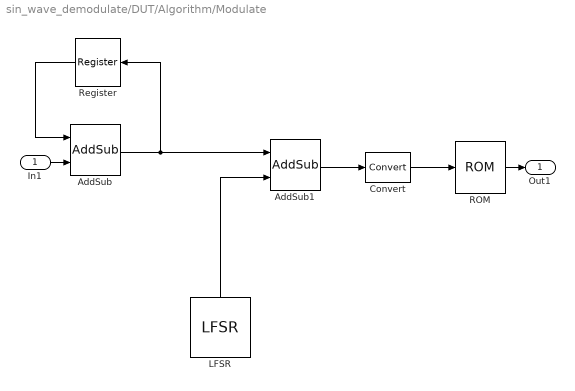
== system sin_wave_demodulate/DUT/Algorithm/Modulate ==
  In1 : Inport
  AddSub : hdlBasic/AddSub  mode=Addition  use_carryin=off  use_carryout=off  en=off  latency=0  precision=User Defined  arith_type=Unsigned  n_bits=14  bin_pt=6  quantization="Round  (unbiased: +/- Inf)"  overflow=Wrap  use_behavioral_HDL=on  hw_selection=Fabric  pipelined=off  use_rpm=on  XmcBlockStatus=1  maskContainerNames=tabcontainer1  block_type=addsub  block_config=sysgen:Addsub_config
  AddSub1 : hdlBasic/AddSub  mode=Addition  use_carryin=off  use_carryout=off  en=off  latency=0  precision=User Defined  arith_type=Unsigned  n_bits=12  bin_pt=4  quantization=Truncate  overflow=Wrap  use_behavioral_HDL=on  hw_selection=Fabric  pipelined=off  use_rpm=on  XmcBlockStatus=1  maskContainerNames=tabcontainer1  block_type=addsub  block_config=sysgen:Addsub_config
  Convert : hdlBasic/Convert  gui_display_data_type=Fixed-point  arith_type=Unsigned  n_bits=8  bin_pt=0  float_type=Single  exp_bits=8  fraction_bits=24  quantization="Round  (unbiased: +/- Inf)"  overflow=Wrap  en=off  latency=1  pipeline=off  XmcBlockStatus=1  maskContainerNames=group2  block_type=convert  block_config=sysgen:Convert_config  block_width=595  block_height=885
  LFSR : hdlBasic/LFSR  lfsr_type=Galois  gate_type=XNOR  n_bits=16  maxpolynomial=on  polynomial='6805'  rst_value='03F'  rst=off  en=off  reloadable_seed=off  input_type=off  output_type=on  arith_type=Unsigned  bin_pt=16  explicit_period=off  period=1/fs  XmcBlockStatus=1  maskContainerNames=tabcontainer1  block_type=lfsr  block_config=sysgen:LFSR_config
  ROM : hdlBasic/ROM  depth=256  initVector=sin(pi*(0:255)/128)  distributed_mem=Block RAM  rst=off  init_reg=0  en=off  latency=1  gui_display_data_type=Fixed-point  arith_type="Signed  (2's comp)"  n_bits=16  bin_pt=15  preci_type=Single  exp_width=8  frac_width=24  optimize=Area  use_rpm=off  simulation_type=fast_sim  XmcBlockStatus=1  maskContainerNames=tabcontainer1  block_type=sprom  block_config=sysgen:SPROM_config
  Register : hdlBasic/Register  init=0  rst=off  en=off  XmcBlockStatus=1  maskContainerNames=tabcontainer1  block_type=register  block_config=sysgen:Register_config
  Out1 : Outport
  wires:
  In1/1 -> AddSub/2
  ROM/1 -> Out1/1
  Convert/1 -> ROM/1
  LFSR/1 -> AddSub1/2
  AddSub/1 -> AddSub1/1, Register/1
  Register/1 -> AddSub/1
  AddSub1/1 -> Convert/1
